simulink model "t5_Punto_3"  (R2021a)
settings: Solver=VariableStepAuto  StartTime=0.0  StopTime=0.04  RelTol=1e-3
libraries: commrandsrc3 x5
settings Model: Creator=HP  LastModifiedBy=HP

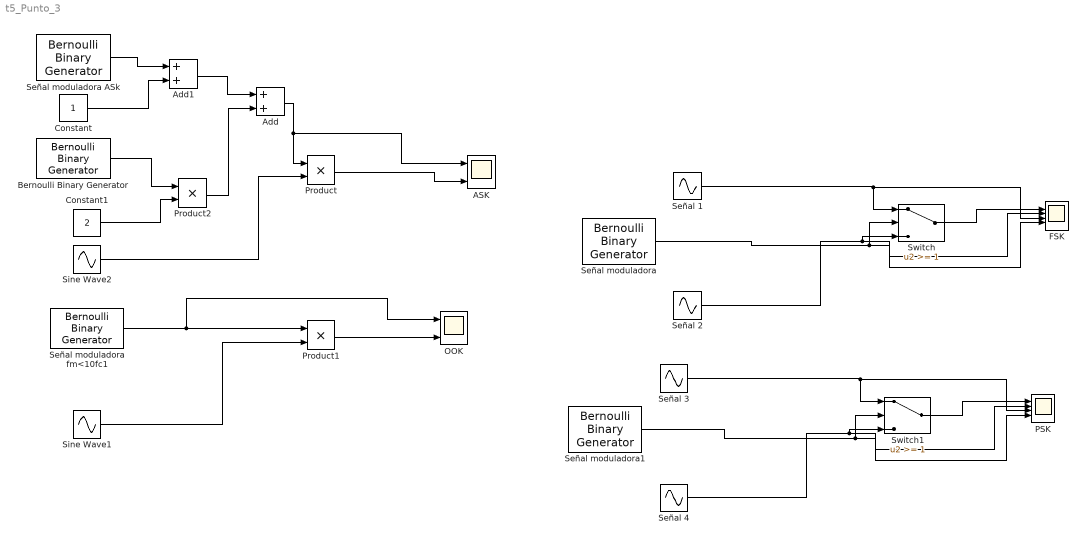
== system t5_Punto_3 ==
  ASK : Scope  NumInputPorts=2
  Add : Sum
  Add1 : Sum
  Bernoulli Binary Generator : commrandsrc3/Bernoulli Binary Generator  ProbabilityOfZero=0.5  SeedSource=Auto  Seed=0  SampleTime=0.01  SamplesPerFrame=1  OutputDataType=double  SimulateUsing=Interpreted execution
  Constant : Constant
  Constant1 : Constant  Value=2
  FSK : Scope  NumInputPorts=4
  OOK : Scope  NumInputPorts=2
  PSK : Scope  NumInputPorts=4
  Product : Product
  Product1 : Product
  Product2 : Product
  Señal 1 : Sin  Amplitude=20  Frequency=150000*2*pi()  SampleTime=0
  Señal 2 : Sin  Amplitude=20  Frequency=300000*2*pi()  SampleTime=0
  Señal 3 : Sin  Amplitude=20  Frequency=1500*2*pi()  SampleTime=0
  Señal 4 : Sin  Amplitude=20  Frequency=1500*2*pi()  Phase=3.66519  SampleTime=0
  Señal moduladora : commrandsrc3/Bernoulli Binary Generator  ProbabilityOfZero=0.5  SeedSource=Parameter  Seed=0  SampleTime=0.00005  SamplesPerFrame=1  OutputDataType=double  SimulateUsing=Interpreted execution
  Señal moduladora ASk : commrandsrc3/Bernoulli Binary Generator  ProbabilityOfZero=0.5  SeedSource=Auto  Seed=0  SampleTime=0.005  SamplesPerFrame=1  OutputDataType=double  SimulateUsing=Interpreted execution
  Señal moduladora fm<10fc1 : commrandsrc3/Bernoulli Binary Generator  ProbabilityOfZero=0.5  SeedSource=Auto  Seed=0  SampleTime=0.001  SamplesPerFrame=1  OutputDataType=double  SimulateUsing=Interpreted execution
  Señal moduladora1 : commrandsrc3/Bernoulli Binary Generator  ProbabilityOfZero=0.5  SeedSource=Parameter  Seed=0  SampleTime=0.001  SamplesPerFrame=1  OutputDataType=double  SimulateUsing=Interpreted execution
  Sine Wave1 : Sin  Amplitude=10  Frequency=2000*2*pi()  SampleTime=0
  Sine Wave2 : Sin  Frequency=1000*2*pi()  SampleTime=0
  Switch : Switch  Threshold=1
  Switch1 : Switch  Threshold=1
  wires:
  Sine Wave1/1 -> Product1/2
  Señal moduladora fm<10fc1/1 -> OOK/1, Product1/1
  Product1/1 -> OOK/2
  Add/1 -> Product/1, ASK/1
  Product/1 -> ASK/2
  Sine Wave2/1 -> Product/2
  Product2/1 -> Add/2
  Señal moduladora ASk/1 -> Add1/1
  Bernoulli Binary Generator/1 -> Product2/1
  Constant1/1 -> Product2/2
  Add1/1 -> Add/1
  Constant/1 -> Add1/2
  Señal moduladora/1 -> FSK/2, Switch/2
  Señal 1/1 -> Switch/1, FSK/3
  Señal 2/1 -> FSK/4, Switch/3
  Switch/1 -> FSK/1
  Señal 3/1 -> Switch1/1, PSK/3
  Señal 4/1 -> PSK/4, Switch1/3
  Switch1/1 -> PSK/1
  Señal moduladora1/1 -> PSK/2, Switch1/2
